simulink model "Electric_ferry_SOC"  (R2021b)
settings: Solver=VariableStepAuto  StartTime=0.0  StopTime=260  RelTol=1
undefined symbols (not defined in the file): ISOC_EF, Pd_EF, QC_ef, R0_ef, V0_ef
libraries: simulink x1
settings Model: Creator=bldha  LastModifiedBy=bldha
settings SolverCC: ZeroCrossAlgorithm=Adaptive
settings DebuggingCC: IgnoredZcDiagnostic=none

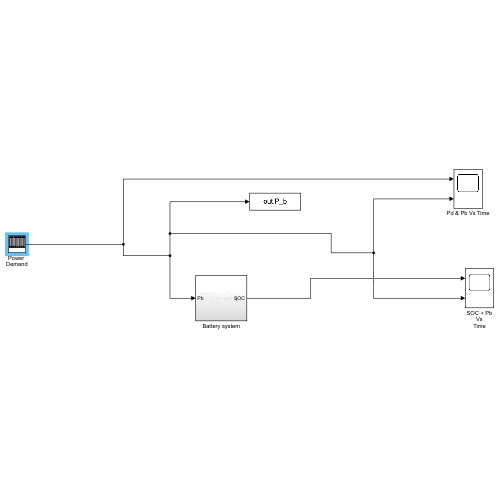
[thumbnail: Simulink's stored preview of the top-level diagram]
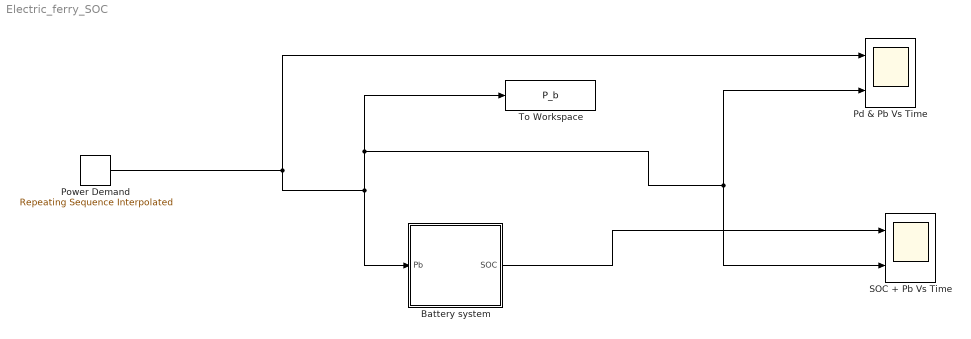
== system Electric_ferry_SOC ==
  Battery system : Subsystem
  Pd & Pb Vs Time : Scope  NumInputPorts=2
  Power Demand : simulink/Sources/Repeating Sequence Interpolated  OutValues=[Pd_EF.pow]  TimeValues=[Pd_EF.time]  LookUpMeth=Interpolation-Use End Values  tsamp=1  OutMin=[]  OutMax=[]  OutDataTypeStr=double  OutputDataTypeScalingMode=double  OutDataType=fixdt(0,8)  OutScaling=2^-10
  SOC + Pb Vs Time : Scope  NumInputPorts=2
  To Workspace : ToWorkspace  VariableName=P_b  SampleTime=-1
  wires:
  Battery system/1(SOC) -> SOC + Pb Vs Time/1
  Power Demand/1 -> Pd & Pb Vs Time/2, SOC + Pb Vs Time/2, To Workspace/1, Battery system/1(Pb), Pd & Pb Vs Time/1

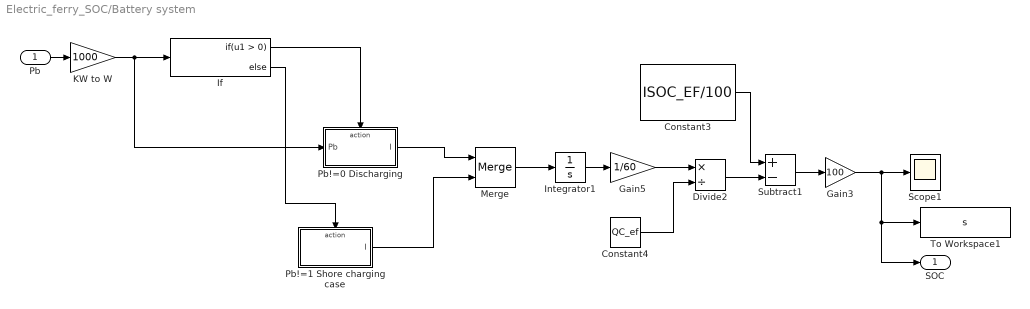
== system Electric_ferry_SOC/Battery system ==
  Pb : Inport
  Constant3 : Constant  Value=ISOC_EF/100
  Constant4 : Constant  Value=QC_ef
  Divide2 : Product  Inputs=*/
  Gain3 : Gain  Gain=100
  Gain5 : Gain  Gain=1/60
  If : If
  Integrator1 : Integrator
  KW to W : Gain  Gain=1000
  Merge : Merge
  Pb!=0 Discharging : Subsystem  TreatAsAtomicUnit=on
  Pb!=1 Shore charging case : Subsystem  TreatAsAtomicUnit=on
  Scope1 : Scope
  Subtract1 : Sum  Inputs=+-
  To Workspace1 : ToWorkspace  VariableName=s  SaveFormat=Structure With Time  SampleTime=-1
  SOC : Outport
  wires:
  Pb/1 -> KW to W/1
  Divide2/1 -> Subtract1/2
  Constant3/1 -> Subtract1/1
  Subtract1/1 -> Gain3/1
  Gain3/1 -> To Workspace1/1, SOC/1, Scope1/1
  Constant4/1 -> Divide2/2
  Gain5/1 -> Divide2/1
  Integrator1/1 -> Gain5/1
  KW to W/1 -> Pb!=0 Discharging/1(Pb), If/1
  If/1 -> Pb!=0 Discharging/Action
  If/2 -> Pb!=1 Shore charging case/Action
  Pb!=0 Discharging/1(I) -> Merge/1
  Pb!=1 Shore charging case/1(I) -> Merge/2
  Merge/1 -> Integrator1/1

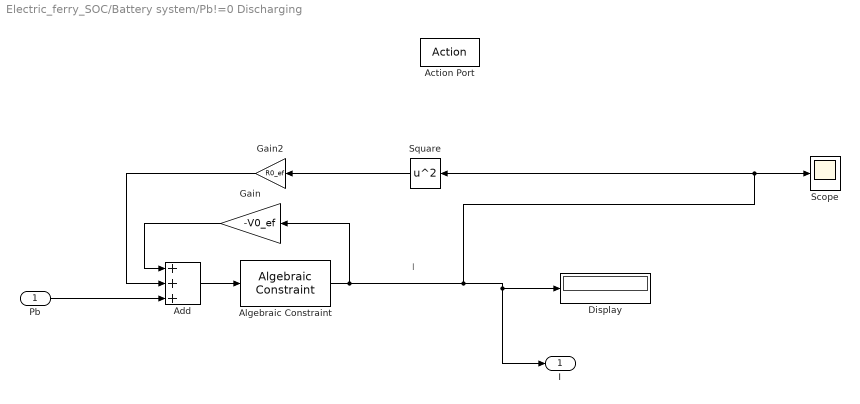
== system Electric_ferry_SOC/Battery system/Pb!=0 Discharging ==
  note: I
  Pb : Inport
  Action Port : ActionPort  ActionPortLabel=if(u1 > 0)
  Add : Sum  Inputs=+++
  Algebraic Constraint : AlgebraicConstraint  InitialGuess=-999999999999
  Display : Display
  Gain : Gain  Gain=-V0_ef
  Gain2 : Gain  Gain=R0_ef
  Scope : Scope
  Square : Math  Operator=square  SaturateOnIntegerOverflow=on
  I : Outport
  wires:
  Square/1 -> Gain2/1
  Algebraic Constraint/1 -> Gain/1, Square/1, Scope/1, I/1, Display/1
  Add/1 -> Algebraic Constraint/1
  Gain2/1 -> Add/2
  Gain/1 -> Add/1
  Pb/1 -> Add/3

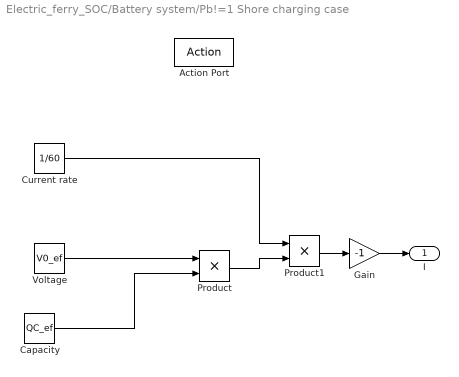
== system Electric_ferry_SOC/Battery system/Pb!=1 Shore charging case ==
  Action Port : ActionPort  ActionPortLabel=else
  Capacity : Constant  Value=QC_ef
  Current rate : Constant  Value=1/60
  Gain : Gain  Gain=-1
  Product : Product
  Product1 : Product
  Voltage : Constant  Value=V0_ef
  I : Outport
  wires:
  Voltage/1 -> Product/1
  Capacity/1 -> Product/2
  Product/1 -> Product1/2
  Current rate/1 -> Product1/1
  Product1/1 -> Gain/1
  Gain/1 -> I/1
